simulink model "Nonlinear_KalmanMPC"  (R2022a)
settings: Solver=FixedStepAuto  StartTime=0.0  StopTime=Tf  FixedStep=Ts  RelTol=1e-3
values from neighbouring files (symbols this model uses):
  D = zeros(size(G2,1),n_y)    [vdp_Koopman.m]
  eta = 0.001    [vdp_MPC.m]
  Ts = ts    [dataset_join.m]    (also in vdp_Koopman.m = 0.01)
undefined symbols (not defined in the file or in its folder): DiscIntNeverNeededParam
libraries: sharedTrackingLibrary x1, mpclib x1
settings Model: Creator=sergiovaneg  LastModifiedBy=sergiovaneg

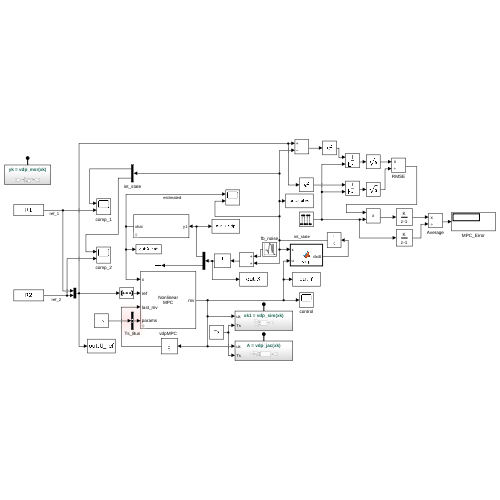
[thumbnail: Simulink's stored preview of the top-level diagram]
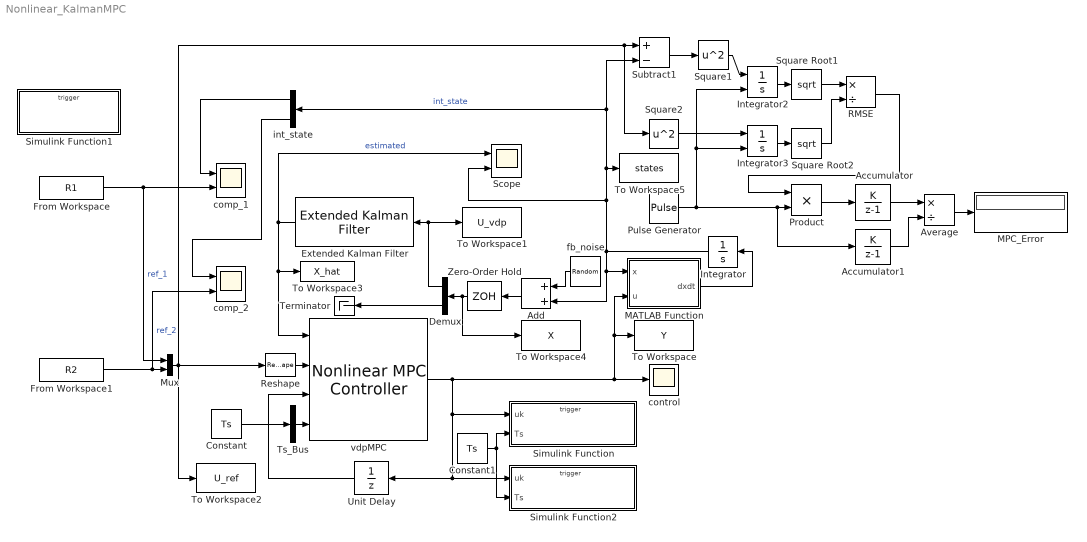
== system Nonlinear_KalmanMPC ==
  Accumulator : DiscreteIntegrator  IntegratorMethod=Accumulation: Forward Euler  InitialCondition=[0;0]  SampleTime=Ts  ICPrevOutput=DiscIntNeverNeededParam  ICPrevScaledInput=DiscIntNeverNeededParam
  Accumulator1 : DiscreteIntegrator  IntegratorMethod=Accumulation: Forward Euler  SampleTime=-1  ICPrevOutput=DiscIntNeverNeededParam  ICPrevScaledInput=DiscIntNeverNeededParam
  Add : Sum
  Average : Product  Inputs=*/
  Constant : Constant  Value=Ts
  Constant1 : Constant  Value=Ts
  Demux : Demux  Outputs=2
  Extended Kalman Filter : sharedTrackingLibrary/Extended Kalman Filter  StateTransitionFcn=vdp_sim  HasStateTransitionJacobianFcn=on  StateTransitionJacobianFcn=vdp_jac  HasAdditiveProcessNoise=Additive  ProcessNoise=eta  HasTimeVaryingProcessNoise=off  HasStateTransitionFcnExtraArgument=0  InitialState=[0;0]  InitialStateCovariance=eta  MeasurementFcn1=vdp_msr  HasMeasurementJacobianFcn1=off  HasMeasurementEnablePort1=off  HasAdditiveMeasurementNoise1=Additive  MeasurementNoise1=eta  HasTimeVaryingMeasurementNoise1=off  HasMeasurementFcnExtraArgument1=0  HasMeasurementWrapping1=off  MeasurementFcn2=myMeasurementFcn  HasMeasurementJacobianFcn2=off  HasMeasurementEnablePort2=off  HasAdditiveMeasurementNoise2=Additive  MeasurementNoise2=1  HasTimeVaryingMeasurementNoise2=off  HasMeasurementFcnExtraArgument2=0  HasMeasurementWrapping2=off  MeasurementFcn3=myMeasurementFcn  HasMeasurementJacobianFcn3=off  HasMeasurementEnablePort3=off  HasAdditiveMeasurementNoise3=Additive  MeasurementNoise3=1  HasTimeVaryingMeasurementNoise3=off  HasMeasurementFcnExtraArgument3=0  HasMeasurementWrapping3=off  MeasurementFcn4=myMeasurementFcn  HasMeasurementJacobianFcn4=off  HasMeasurementEnablePort4=off  HasAdditiveMeasurementNoise4=Additive  MeasurementNoise4=1  HasTimeVaryingMeasurementNoise4=off  HasMeasurementFcnExtraArgument4=0  HasMeasurementWrapping4=off  MeasurementFcn5=myMeasurementFcn  HasMeasurementJacobianFcn5=off  HasMeasurementEnablePort5=off  HasAdditiveMeasurementNoise5=Additive  MeasurementNoise5=1  HasTimeVaryingMeasurementNoise5=off  HasMeasurementFcnExtraArgument5=0  HasMeasurementWrapping5=off  EnableMultirate=off  StateTransitionFcnSampleTime=1  MeasurementFcn1SampleTime=1  MeasurementFcn2SampleTime=1  MeasurementFcn3SampleTime=1  MeasurementFcn4SampleTime=1  MeasurementFcn5SampleTime=1  UseCurrentEstimator=on  OutputStateCovariance=off  DataType=double  SampleTime=Ts  NumberOfMeasurements=1
      settings: SourceProductBaseCode=TF,AE,PW,CT,DR,ID,LP,NV,AR,RO,RR,UV,VE
  From Workspace : FromWorkspace  VariableName=R1
  From Workspace1 : FromWorkspace  VariableName=R2
  Integrator : Integrator  InitialCondition=[0;0]
  Integrator2 : Integrator  ExternalReset=falling  InitialCondition=[0;0]
  Integrator3 : Integrator  ExternalReset=falling  InitialCondition=[eps;eps]
  MATLAB Function : MATLAB Function  TreatAsAtomicUnit=on
  MPC_Error : Display
  Mux : Mux  Inputs=2
  Product : Product
  Pulse Generator : DiscretePulseGenerator  Period=10/Ts  SampleTime=Ts
  RMSE : Product  Inputs=*/
  Reshape : Reshape  OutputDimensionality=Row vector (2-D)
  Scope : Scope  NumInputPorts=2
  Simulink Function : Subsystem  TreatAsAtomicUnit=on
  Simulink Function1 : Subsystem  TreatAsAtomicUnit=on
  Simulink Function2 : Subsystem  TreatAsAtomicUnit=on
  Square Root1 : Sqrt
  Square Root2 : Sqrt
  Square1 : Math  Operator=square
  Square2 : Math  Operator=square
  Subtract1 : Sum  Inputs=+-
  Terminator : Terminator
  To Workspace : ToWorkspace  VariableName=Y  SampleTime=Ts
      settings: Save2DSignal=2-D array (concatenate along first dimension)
  To Workspace1 : ToWorkspace  VariableName=U_vdp  SampleTime=Ts
      settings: Save2DSignal=2-D array (concatenate along first dimension)
  To Workspace2 : ToWorkspace  VariableName=U_ref  SampleTime=Ts
      settings: Save2DSignal=2-D array (concatenate along first dimension)
  To Workspace3 : ToWorkspace  VariableName=X_hat  SampleTime=Ts
      settings: Save2DSignal=2-D array (concatenate along first dimension)
  To Workspace4 : ToWorkspace  VariableName=X  SampleTime=Ts
      settings: Save2DSignal=2-D array (concatenate along first dimension)
  To Workspace5 : ToWorkspace  VariableName=states  SampleTime=Ts
      settings: Save2DSignal=2-D array (concatenate along first dimension)
  Ts_Bus : BusCreator  Inputs=1  OutDataTypeStr=Bus: Ts_Bus  NonVirtualBus=on
      settings: InheritFromInputs=off
  Unit Delay : UnitDelay  SampleTime=-1  HasFrameUpgradeWarning=on
  Zero-Order Hold : ZeroOrderHold  SampleTime=Ts
  comp_1 : Scope  NumInputPorts=2
  comp_2 : Scope  NumInputPorts=2
  control : Scope
  fb_noise : RandomNumber  Variance=eta  Seed=[2;3]  SampleTime=Ts
  int_state : Demux  Outputs=2
  vdpMPC : mpclib/Nonlinear MPC Controller  nlmpcobj=nlobj  UseObjectTs=on  UseMEX=off  md_enabled=off  mvtarget_enabled=off  param_enabled=on  cost_enabled=off  mvseq_enabled=off  stateseq_enabled=off  ovseq_enabled=off  slack_enabled=off  status_enabled=off  ov_min=off  ov_max=off  mv_min=off  mv_max=off  mvrate_min=off  mvrate_max=off  state_min=off  state_max=off  ov_weight=off  mv_weight=off  mvrate_weight=off  ecr_weight=off  nlp_initialize=off
  wires:
  int_state/1 -> comp_1/1
  fb_noise/1 -> Add/1
  Reshape/1 -> vdpMPC/2
  vdpMPC/1 -> MATLAB Function/2(u), To Workspace/1, control/1, Simulink Function2/1(uk), Unit Delay/1, Simulink Function/1(uk)
  Constant/1 -> Ts_Bus/1
  Integrator/1 -> To Workspace5/1, Subtract1/2, int_state/1, Scope/2, Add/2, MATLAB Function/1(x)  "int_state"
  From Workspace1/1 -> comp_2/2, Mux/2  "ref_2"
  Unit Delay/1 -> vdpMPC/3
  int_state/2 -> comp_2/1
  MATLAB Function/1(dxdt) -> Integrator/1
  Mux/1 -> Square2/1, Subtract1/1, To Workspace2/1, Reshape/1
  Ts_Bus/1 -> vdpMPC/4
  Demux/1 -> Extended Kalman Filter/1, To Workspace1/1
  Demux/2 -> Terminator/1
  Extended Kalman Filter/1 -> vdpMPC/1, To Workspace3/1, Scope/1  "estimated"
  Zero-Order Hold/1 -> To Workspace4/1, Demux/1
  Add/1 -> Zero-Order Hold/1
  Constant1/1 -> Simulink Function/2(Ts), Simulink Function2/2(Ts)
  From Workspace/1 -> comp_1/2, Mux/1  "ref_1"
  Square Root2/1 -> RMSE/2
  Product/1 -> Accumulator/1
  Integrator3/1 -> Square Root2/1
  Accumulator/1 -> Average/1
  RMSE/1 -> Product/1
  Accumulator1/1 -> Average/2
  Average/1 -> MPC_Error/1
  Square2/1 -> Integrator3/1
  Square Root1/1 -> RMSE/1
  Integrator2/1 -> Square Root1/1
  Square1/1 -> Integrator2/1
  Pulse Generator/1 -> Integrator2/2, Integrator3/2, Accumulator1/1, Product/2
  Subtract1/1 -> Square1/1

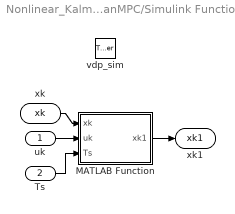
== system Nonlinear_KalmanMPC/Simulink Function ==
  uk : Inport
  Ts : Inport  Port=2
  vdp_sim : TriggerPort  TriggerType=function-call  IsSimulinkFunction=on  FunctionName=vdp_sim  FunctionVisibility=scoped  VariantControl=(inherit)
  MATLAB Function : MATLAB Function  TreatAsAtomicUnit=on
  xk : ArgIn  DisableCoverage=on  PortDimensions=2  ArgumentName=xk
  xk1 : ArgOut  DisableCoverage=on  PortDimensions=2  ArgumentName=xk1
  wires:
  xk/1 -> MATLAB Function/1(xk)
  MATLAB Function/1(xk1) -> xk1/1
  uk/1 -> MATLAB Function/2(uk)
  Ts/1 -> MATLAB Function/3(Ts)

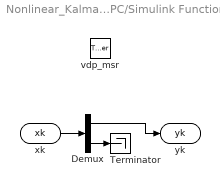
== system Nonlinear_KalmanMPC/Simulink Function1 ==
  vdp_msr : TriggerPort  TriggerType=function-call  IsSimulinkFunction=on  FunctionName=vdp_msr  FunctionVisibility=scoped  VariantControl=(inherit)
  Demux : Demux  Outputs=2
  Terminator : Terminator
  xk : ArgIn  DisableCoverage=on  PortDimensions=2  ArgumentName=xk
  yk : ArgOut  DisableCoverage=on  ArgumentName=yk
  wires:
  Demux/2 -> Terminator/1
  xk/1 -> Demux/1
  Demux/1 -> yk/1

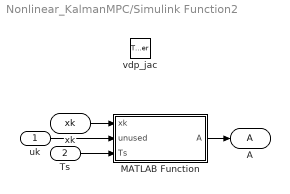
== system Nonlinear_KalmanMPC/Simulink Function2 ==
  uk : Inport
  Ts : Inport  Port=2
  vdp_jac : TriggerPort  TriggerType=function-call  IsSimulinkFunction=on  FunctionName=vdp_jac  FunctionVisibility=scoped  VariantControl=(inherit)
  MATLAB Function : MATLAB Function  TreatAsAtomicUnit=on
  xk : ArgIn  DisableCoverage=on  PortDimensions=2  ArgumentName=xk
  A : ArgOut  DisableCoverage=on  PortDimensions=[2 2]  ArgumentName=A
  wires:
  xk/1 -> MATLAB Function/1(xk)
  MATLAB Function/1(A) -> A/1
  uk/1 -> MATLAB Function/2(unused)
  Ts/1 -> MATLAB Function/3(Ts)

== matlab function Nonlinear_KalmanMPC/Simulink Function/MATLAB Function ==
  data: xk input; xk1 output; uk input; Ts input
function xk1 = vdp(xk,uk,Ts)
    M = 10;

    delta = Ts/M;
    xk1 = xk;
    for ct=1:M
        xk1 = xk1+delta*vdp_CT0(xk,uk);
    end
end

== matlab function Nonlinear_KalmanMPC/MATLAB Function ==
  data: x input; u input; dxdt output
function dxdt = vdp(x,u)
    dxdt = zeros(2,1);
    dxdt(1) = 2*x(2);
    dxdt(2) = -0.8*x(1)+2*x(2)-10*(x(1)^2)*x(2)+u;

== matlab function Nonlinear_KalmanMPC/Simulink Function2/MATLAB Function ==
  data: xk input; A output; unused input; Ts input
function A = fcn(xk,~,Ts)
    A=[1,2*Ts;
        Ts*(-0.8-20*xk(1)*xk(2)),1+Ts*(2-xk(1)^2)];
end
